simulink model "exp12"  (R2021b)
settings: Solver=VariableStepAuto  StartTime=0.0  StopTime=10  RelTol=1e-3
undefined symbols (not defined in the file): a, b, c, d, e
libraries: simulink_extras x1, spspowerguiLib x1
settings Model: Creator=amans  LastModifiedBy=amans

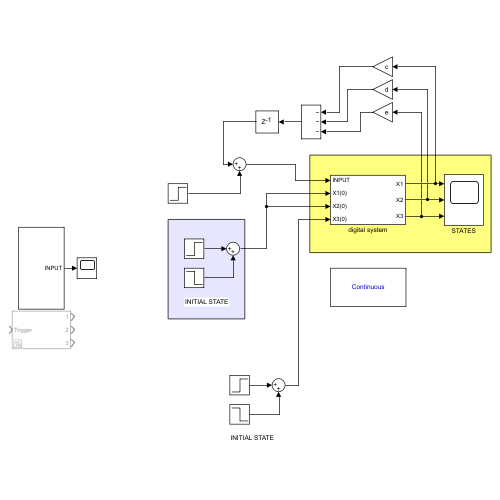
[thumbnail: Simulink's stored preview of the top-level diagram]
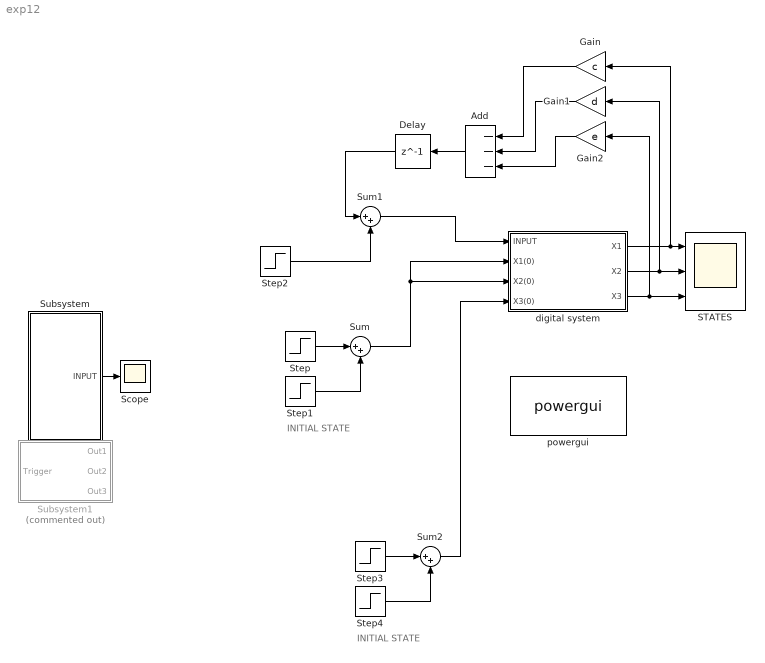
== system exp12 ==
  note: INITIAL STATE
  note: INITIAL STATE
  Add : Sum  Inputs=---
  Delay : Delay  DelayLength=1
  Gain : Gain  Gain=c
  Gain1 : Gain  Gain=d
  Gain2 : Gain  Gain=e
  STATES : Scope  NumInputPorts=3
  Scope : Scope
  Step : Step  Time=0.5  SampleTime=0
  Step1 : Step  Time=1.5  After=-1  SampleTime=0
  Step2 : Step  Time=1.5  After=4  SampleTime=0
  Step3 : Step  Time=0.5  After=2  SampleTime=0
  Step4 : Step  Time=1.5  After=-2  SampleTime=0
  Subsystem : Subsystem
  Subsystem1 : Subsystem  Commented=on
  Sum : Sum  Inputs=|++
  Sum1 : Sum  Inputs=|++
  Sum2 : Sum  Inputs=|++
  digital system : Subsystem
  powergui : spspowerguiLib/powergui  Priority=1  SimulationMode=Continuous  SampleTime=50e-6  frequency=60  Iterations=50  frequencyindice=60  Pbase=100e6  ErrMax=1e-4  UnitsV=kV  UnitsW=MW  buscounter=0  FunctionMessages=off  echomessages=off  EnableUseOfTLC=off  CurrentSourceSwitches=off  DisableSnubberDevices=off  DisableRonSwitches=off  DisableVfSwitches=off  DisplayEquations=off  AutomaticDiscreteSolvers=off  SolverType=Tustin/Backward Euler (TBE)  Interpol=off  ExternalGateDelay=off  methode=off  Ts=100  x0status=blocks  SPID=on  SwTol=0  HookPort=off  NonlinearTolerance=1e-4  nMaxIteration=100  ContinueOnMaxIteration=off  RestoreLinks=warning  ResistiveCurrentMeasurement=off  Frange=[0:2:500]  Ylog=off  Xlog=on  ShowGrid=off  save=off  variable=ZData  structure=0  ZoomFFT=off  StartTime=0.0  cycles=1  DisplayStyle=1  fundamental=60  FreqAxis=off  MaxFrequency=1000  frequencyindicesteady=1  RmsSteady=1  display=off
  wires:
  digital system/1(X1) -> Gain/1, STATES/1
  digital system/2(X2) -> STATES/2, Gain1/1
  digital system/3(X3) -> Gain2/1, STATES/3
  Step/1 -> Sum/1
  Step1/1 -> Sum/2
  Sum/1 -> digital system/3(X2(0)), digital system/2(X1(0))
  Subsystem/1(INPUT) -> Scope/1
  Add/1 -> Delay/1
  Gain/1 -> Add/1
  Gain1/1 -> Add/2
  Gain2/1 -> Add/3
  Delay/1 -> Sum1/1
  Sum1/1 -> digital system/1(INPUT)
  Step2/1 -> Sum1/2
  Step4/1 -> Sum2/2
  Step3/1 -> Sum2/1
  Sum2/1 -> digital system/4(X3(0))

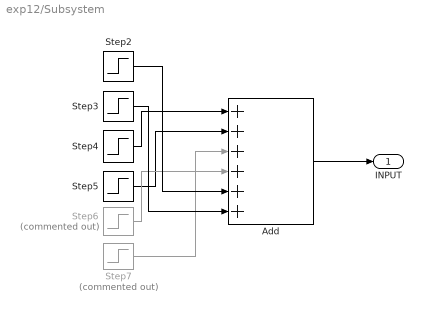
== system exp12/Subsystem ==
  Add : Sum  Inputs=++++++
  Step2 : Step  Time=1.5  After=-1  SampleTime=0
  Step3 : Step  Time=2.5  SampleTime=0
  Step4 : Step  Time=2.5  After=-10  SampleTime=0
  Step5 : Step  Time=3.5  After=10  SampleTime=0
  Step6 : Step  Commented=on  Time=3.5  After=-0.7  SampleTime=0
  Step7 : Step  Commented=on  Time=4.5  After=0.7  SampleTime=0
  INPUT : Outport
  wires:
  Add/1 -> INPUT/1
  Step4/1 -> Add/1
  Step5/1 -> Add/2
  Step7/1 -> Add/3
  Step6/1 -> Add/4
  Step2/1 -> Add/5
  Step3/1 -> Add/6

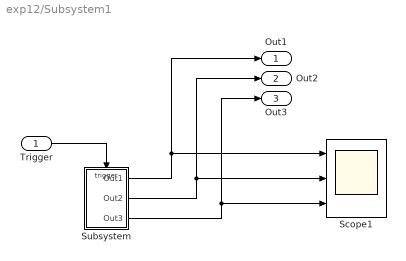
== system exp12/Subsystem1 ==
  Trigger : Inport
  Scope1 : Scope  NumInputPorts=3
  Subsystem : Subsystem
  Out1 : Outport
  Out2 : Outport  Port=2
  Out3 : Outport  Port=3
  wires:
  Subsystem/1(Out1) -> Out1/1, Scope1/1
  Trigger/1 -> Subsystem/Trigger
  Subsystem/2(Out2) -> Out2/1, Scope1/2
  Subsystem/3(Out3) -> Out3/1, Scope1/3

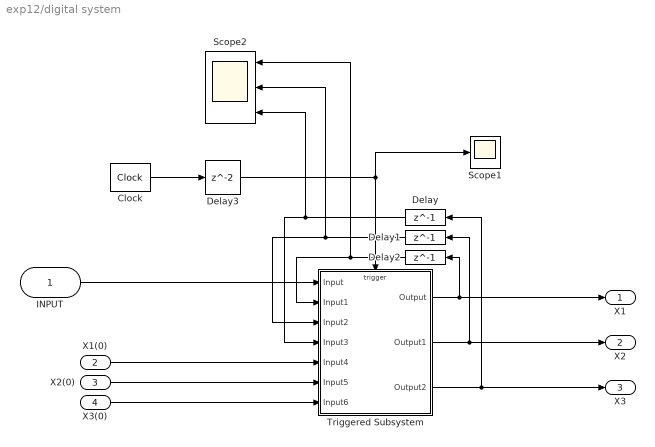
== system exp12/digital system ==
  INPUT : Inport
  X1(0) : Inport  Port=2
  X2(0) : Inport  Port=3
  X3(0) : Inport  Port=4
  Clock : simulink_extras/Flip Flops/Clock  period=1
  Delay : Delay  DelayLength=1
  Delay1 : Delay  DelayLength=1
  Delay2 : Delay  DelayLength=1
  Delay3 : Delay
  Scope1 : Scope
  Scope2 : Scope  NumInputPorts=3
  Triggered Subsystem : Subsystem  TreatAsAtomicUnit=on
  X1 : Outport
  X2 : Outport  Port=2
  X3 : Outport  Port=3
  wires:
  Triggered Subsystem/1(Output) -> Delay2/1, X1/1
  X1(0)/1 -> Triggered Subsystem/5(Input4)
  X2(0)/1 -> Triggered Subsystem/6(Input5)
  X3(0)/1 -> Triggered Subsystem/7(Input6)
  Triggered Subsystem/3(Output2) -> Delay/1, X3/1
  Triggered Subsystem/2(Output1) -> Delay1/1, X2/1
  Delay2/1 -> Triggered Subsystem/2(Input1), Scope2/1
  Delay/1 -> Scope2/3, Triggered Subsystem/4(Input3)
  Clock/1 -> Delay3/1
  Delay1/1 -> Triggered Subsystem/3(Input2), Scope2/2
  Delay3/1 -> Scope1/1, Triggered Subsystem/Trigger
  INPUT/1 -> Triggered Subsystem/1(Input)

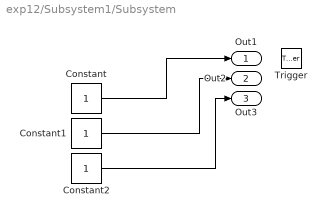
== system exp12/Subsystem1/Subsystem ==
  Trigger : TriggerPort  VariantControl=(inherit)  PortDimensions=1
  Constant : Constant
  Constant1 : Constant
  Constant2 : Constant
  Out1 : Outport
  Out2 : Outport  Port=2
  Out3 : Outport  Port=3
  wires:
  Constant1/1 -> Out2/1
  Constant2/1 -> Out3/1
  Constant/1 -> Out1/1

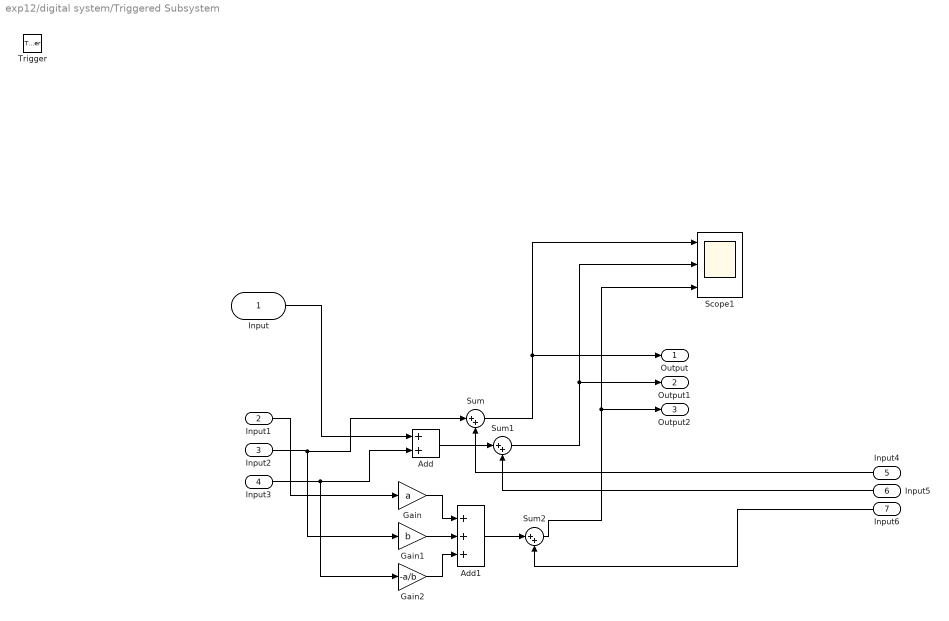
== system exp12/digital system/Triggered Subsystem ==
  Input : Inport
  Input1 : Inport  Port=2
  Input2 : Inport  Port=3
  Input3 : Inport  Port=4
  Input4 : Inport  Port=5
  Input5 : Inport  Port=6
  Input6 : Inport  Port=7
  Trigger : TriggerPort  VariantControl=(inherit)
  Add : Sum
  Add1 : Sum  Inputs=+++
  Gain : Gain  Gain=a
  Gain1 : Gain  Gain=b
  Gain2 : Gain  Gain=-a/b
  Scope1 : Scope  NumInputPorts=3
  Sum : Sum  Inputs=|++
  Sum1 : Sum  Inputs=|++
  Sum2 : Sum  Inputs=|++
  Output : Outport
  Output1 : Outport  Port=2
  Output2 : Outport  Port=3
  wires:
  Input6/1 -> Sum2/2
  Input4/1 -> Sum/2
  Input1/1 -> Gain/1
  Input2/1 -> Sum/1, Gain1/1
  Input/1 -> Add/1
  Input3/1 -> Gain2/1, Add/2
  Sum/1 -> Output/1, Scope1/1
  Gain/1 -> Add1/1
  Sum2/1 -> Output2/1, Scope1/3
  Sum1/1 -> Output1/1, Scope1/2
  Input5/1 -> Sum1/2
  Gain2/1 -> Add1/3
  Add/1 -> Sum1/1
  Add1/1 -> Sum2/1
  Gain1/1 -> Add1/2
